simulink library "vectorNormalizer_ul"  (R2018b)
settings: Solver=VariableStepAuto  StartTime=0.0  StopTime=10.0  RelTol=1e-3
settings Model: Creator=James Reed  LastModifiedBy=mcobb

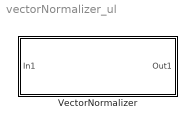
== system vectorNormalizer_ul ==
  "VectorNormalizer " : Subsystem

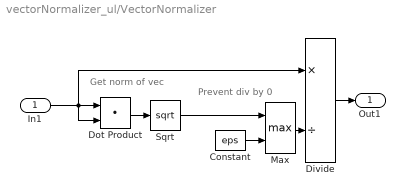
== system vectorNormalizer_ul/VectorNormalizer  ==
  note: Get norm of vec
  note: Prevent div by 0
  In1 : Inport
  Constant : Constant  Value=eps
  Divide : Product  Inputs=*/
  Dot Product : DotProduct  InputSameDT=on  OutDataTypeStr=Inherit: Inherit via internal rule
  Max : MinMax  Function=max  Inputs=2
  Sqrt : Sqrt  SaturateOnIntegerOverflow=on
  Out1 : Outport
  wires:
  Sqrt/1 -> Max/1
  In1/1 -> Divide/1, Dot Product/2, Dot Product/1
  Dot Product/1 -> Sqrt/1
  Divide/1 -> Out1/1
  Max/1 -> Divide/2
  Constant/1 -> Max/2
